simulink model "comparaCascataFF"  (R2017a)
settings: Solver=VariableStepAuto  StartTime=0.0  StopTime=50  RelTol=1e-3
settings Model: Creator=julia  LastModifiedBy=julia

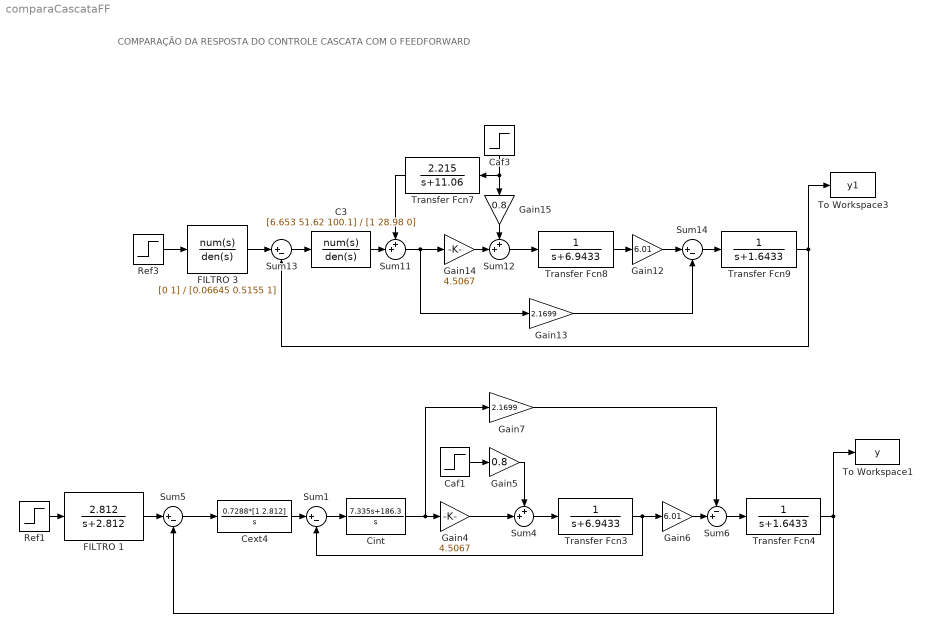
== system comparaCascataFF ==
  note: COMPARAÇÃO DA RESPOSTA DO CONTROLE CASCATA COM O FEEDFORWARD
  C3 : TransferFcn  Numerator=[6.653 51.62 100.1]  Denominator=[1 28.98 0]
  Caf1 : Step  Time=20  After=0.1  SampleTime=0
  Caf3 : Step  Time=20  After=0.1  SampleTime=0
  Cext4 : TransferFcn  Numerator=0.7288*[1 2.812]  Denominator=[1 0]
  Cint : TransferFcn  Numerator=[7.335 186.3]  Denominator=[1 0]
  FILTRO 1 : TransferFcn  Numerator=[2.812]  Denominator=[1 2.812]
  FILTRO 3 : TransferFcn  Numerator=[0 1]  Denominator=[0.06645 0.5155 1]
  Gain12 : Gain  Gain=6.01
  Gain13 : Gain  Gain=2.1699
  Gain14 : Gain  Gain=4.5067
  Gain15 : Gain  Gain=0.8
  Gain4 : Gain  Gain=4.5067
  Gain5 : Gain  Gain=0.8
  Gain6 : Gain  Gain=6.01
  Gain7 : Gain  Gain=2.1699
  Ref1 : Step  Time=0  After=0.1  SampleTime=0
  Ref3 : Step  Time=0  After=0.1  SampleTime=0
  Sum{1,5,13..14} (4 alike) : Sum  Inputs=|+-
  Sum11 : Sum  Inputs=++|
  Sum12 : Sum  Inputs=++|
  Sum4 : Sum  Inputs=++|
  Sum6 : Sum  Inputs=-+|
  To Workspace1 : ToWorkspace  VariableName=y  SaveFormat=Timeseries  SampleTime=-1
  To Workspace3 : ToWorkspace  VariableName=y1  SaveFormat=Timeseries  SampleTime=-1
  Transfer Fcn3 : TransferFcn  Denominator=[1 6.9433]
  Transfer Fcn4 : TransferFcn  Denominator=[1 1.6433]
  Transfer Fcn7 : TransferFcn  Numerator=[0 2.215]  Denominator=[1 11.06]
  Transfer Fcn8 : TransferFcn  Denominator=[1 6.9433]
  Transfer Fcn9 : TransferFcn  Denominator=[1 1.6433]
  wires:
  C3/1 -> Sum11/2
  Transfer Fcn7/1 -> Sum11/1
  Sum11/1 -> Gain13/1, Gain14/1
  Caf3/1 -> Transfer Fcn7/1, Gain15/1
  Sum14/1 -> Transfer Fcn9/1
  Gain12/1 -> Sum14/1
  Sum13/1 -> C3/1
  Ref3/1 -> FILTRO 3/1
  FILTRO 3/1 -> Sum13/1
  Gain13/1 -> Sum14/2
  Gain14/1 -> Sum12/2
  Sum12/1 -> Transfer Fcn8/1
  Gain15/1 -> Sum12/1
  Transfer Fcn8/1 -> Gain12/1
  Transfer Fcn9/1 -> To Workspace3/1, Sum13/2
  Ref1/1 -> FILTRO 1/1
  Cint/1 -> Gain7/1, Gain4/1
  Sum6/1 -> Transfer Fcn4/1
  Gain7/1 -> Sum6/1
  FILTRO 1/1 -> Sum5/1
  Gain5/1 -> Sum4/1
  Sum5/1 -> Cext4/1
  Transfer Fcn4/1 -> To Workspace1/1, Sum5/2
  Sum1/1 -> Cint/1
  Transfer Fcn3/1 -> Gain6/1, Sum1/2
  Gain4/1 -> Sum4/2
  Cext4/1 -> Sum1/1
  Sum4/1 -> Transfer Fcn3/1
  Caf1/1 -> Gain5/1
  Gain6/1 -> Sum6/2
